simulink model "Lab5"  (R2023b)
settings: Solver=VariableStepAuto  StartTime=0.0  StopTime=10.0  RelTol=1e-3
settings Model: Creator=eevaa  LastModifiedBy=chayn

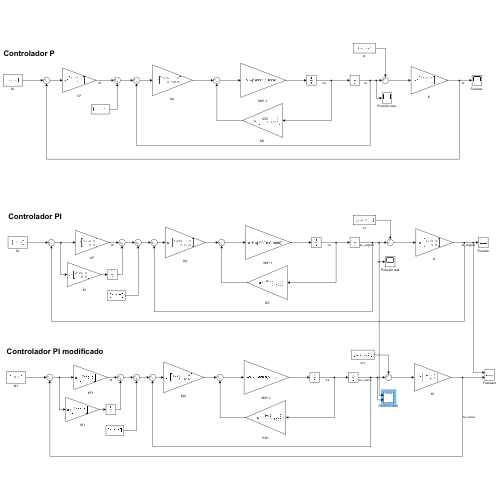
[thumbnail: Simulink's stored preview of the top-level diagram]
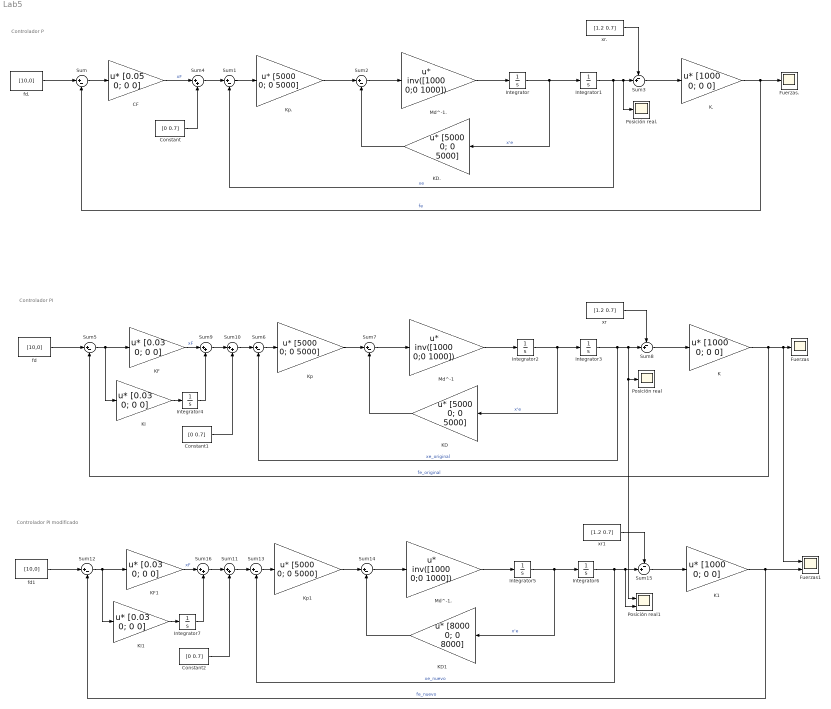
== system Lab5 ==
  note: Controlador P
  note: Controlador PI
  note: Controlador PI modificado
  CF : Gain  Gain=[0.05 0; 0 0]  Multiplication=Matrix(u*K)
  Constant : Constant  Value=[0 0.7]
  Constant1 : Constant  Value=[0 0.7]
  Constant2 : Constant  Value=[0 0.7]
  Fuerzas : Scope
  Fuerzas. : Scope
  Fuerzas1 : Scope  NumInputPorts=2
  Integrator{,2,4..5,7} (5 alike) : Integrator
  Integrator1 : Integrator  InitialCondition=[1.3 0.7]
  Integrator3 : Integrator  InitialCondition=[1.3 0.7]
  Integrator6 : Integrator  InitialCondition=[1.3 0.7]
  K : Gain  Gain=[1000 0; 0 0]  Multiplication=Matrix(u*K)
  K. : Gain  Gain=[1000 0; 0 0]  Multiplication=Matrix(u*K)
  K1 : Gain  Gain=[1000 0; 0 0]  Multiplication=Matrix(u*K)
  KD : Gain  Gain=[5000 0; 0 5000]  Multiplication=Matrix(u*K)
  KD. : Gain  Gain=[5000 0; 0 5000]  Multiplication=Matrix(u*K)
  KD1 : Gain  Gain=[8000 0; 0 8000]  Multiplication=Matrix(u*K)
  KF : Gain  Gain=[0.03 0; 0 0]  Multiplication=Matrix(u*K)
  KF1 : Gain  Gain=[0.03 0; 0 0]  Multiplication=Matrix(u*K)
  KI : Gain  Gain=[0.03 0; 0 0]  Multiplication=Matrix(u*K)
  KI1 : Gain  Gain=[0.03 0; 0 0]  Multiplication=Matrix(u*K)
  Kp : Gain  Gain=[5000 0; 0 5000]  Multiplication=Matrix(u*K)
  Kp. : Gain  Gain=[5000 0; 0 5000]  Multiplication=Matrix(u*K)
  Kp1 : Gain  Gain=[5000 0; 0 5000]  Multiplication=Matrix(u*K)
  Md^-1 : Gain  Gain=inv([1000 0;0 1000])  Multiplication=Matrix(u*K)
  Md^-1, : Gain  Gain=inv([1000 0;0 1000])  Multiplication=Matrix(u*K)
  Md^-1. : Gain  Gain=inv([1000 0;0 1000])  Multiplication=Matrix(u*K)
  Posición real : Scope
  Posición real. : Scope
  Posición real1 : Scope  NumInputPorts=2
  Sum{,1..2,5..7,12..14} (9 alike) : Sum  Inputs=|+-
  Sum{4,9..11,16} (5 alike) : Sum  Inputs=|++
  Sum15 : Sum  Inputs=-+|
  Sum3 : Sum  Inputs=-+|
  Sum8 : Sum  Inputs=-+|
  fd : Constant  Value=[10,0]
  fd. : Constant  Value=[10,0]
  fd1 : Constant  Value=[10,0]
  xr : Constant  Value=[1.2 0.7]
  xr. : Constant  Value=[1.2 0.7]
  xr1 : Constant  Value=[1.2 0.7]
  wires:
  fd./1 -> Sum/1
  Sum/1 -> CF/1
  Sum1/1 -> Kp./1
  Kp./1 -> Sum2/1
  Sum2/1 -> Md^-1./1
  Md^-1./1 -> Integrator/1
  Integrator/1 -> KD./1, Integrator1/1  "x'e"
  KD./1 -> Sum2/2
  Integrator1/1 -> Sum1/2, Posición real./1, Sum3/2  "xe"
  xr./1 -> Sum3/1
  Sum3/1 -> K./1
  K./1 -> Sum/2, Fuerzas./1  "fe"
  K/1 -> Fuerzas1/1, Fuerzas/1, Sum5/2  "fe_original"
  Integrator4/1 -> Sum9/2
  Integrator3/1 -> Posición real1/1, Posición real/1, Sum8/2, Sum6/2  "xe_original"
  xr/1 -> Sum8/1
  KD/1 -> Sum7/2
  Sum7/1 -> Md^-1/1
  Integrator2/1 -> KD/1, Integrator3/1  "x'e"
  Md^-1/1 -> Integrator2/1
  Sum5/1 -> KI/1, KF/1
  Sum6/1 -> Kp/1
  fd/1 -> Sum5/1
  Kp/1 -> Sum7/1
  Sum8/1 -> K/1
  KF/1 -> Sum9/1  "xF"
  KI/1 -> Integrator4/1
  Constant1/1 -> Sum10/2
  Sum10/1 -> Sum6/1
  Sum9/1 -> Sum10/1
  Constant/1 -> Sum4/2
  CF/1 -> Sum4/1  "xF"
  Sum4/1 -> Sum1/1
  Sum14/1 -> Md^-1,/1
  Integrator5/1 -> KD1/1, Integrator6/1  "x'e"
  Sum16/1 -> Sum11/1
  Sum11/1 -> Sum13/1
  Sum15/1 -> K1/1
  Md^-1,/1 -> Integrator5/1
  KD1/1 -> Sum14/2
  KI1/1 -> Integrator7/1
  Kp1/1 -> Sum14/1
  Sum13/1 -> Kp1/1
  KF1/1 -> Sum16/1  "xF"
  Integrator6/1 -> Posición real1/2, Sum15/2, Sum13/2  "xe_nuevo"
  Sum12/1 -> KI1/1, KF1/1
  Integrator7/1 -> Sum16/2
  Constant2/1 -> Sum11/2
  K1/1 -> Sum12/2, Fuerzas1/2  "fe_nuevo"
  fd1/1 -> Sum12/1
  xr1/1 -> Sum15/1
